simulink model "vdp_1_mode"  (R2020a)
settings: Solver=VariableStepAuto  StartTime=0.0  StopTime=60  RelTol=1e-3
libraries: dspsnks4 x1
settings Model: EnablePacing=on  Creator=Dinh-Viet-Toan  LastModifiedBy=Dinh-Viet-Toan

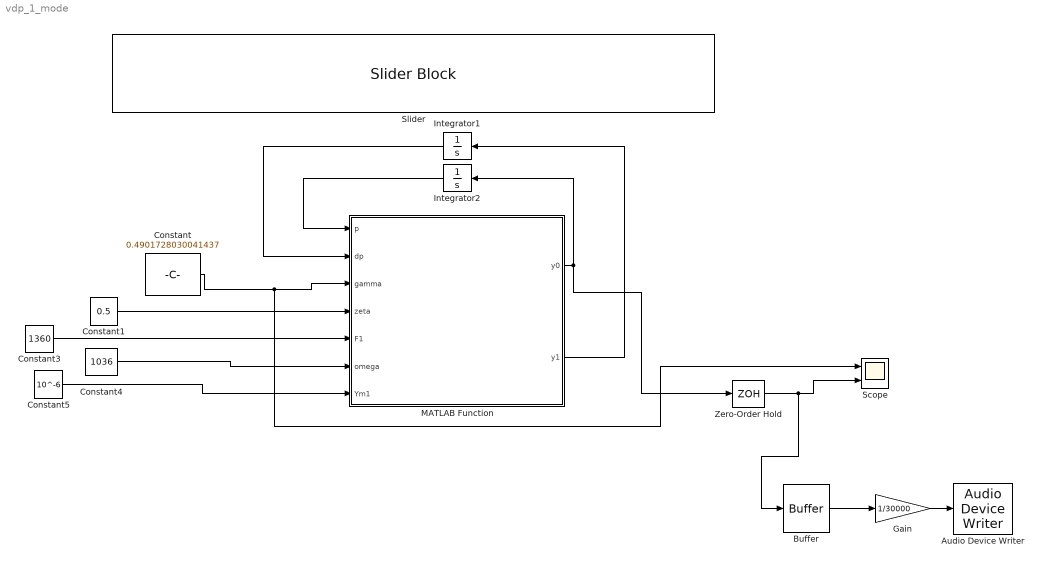
== system vdp_1_mode ==
  Audio Device Writer : dspsnks4/Audio Device Writer  Driver=DirectSound  Device=Default  InheritSampleRate=on  SampleRate=44100  BitDepth=16-bit integer  BufferSize=4096  NumBuffers=10  DefaultOutputChannelMapping=on  OutputChannelMapping=1:2  OutputNumUnderrunSamples=off  DriverIdx=1  DeviceWarnFlag=''
  Buffer : Buffer  N=10000  V=1024  OutputFrames=off
  Constant : Constant  Value=0.4901728030041437
  Constant1 : Constant  Value=0.5
  Constant3 : Constant  Value=1360
  Constant4 : Constant  Value=1036
  Constant5 : Constant  Value=10^-6
  Gain : Gain  Gain=1/30000
  Integrator1 : Integrator
  Integrator2 : Integrator  InitialCondition=0.01
  MATLAB Function : MATLAB Function  TreatAsAtomicUnit=on
  Scope : Scope  NumInputPorts=2
  Slider : SliderBlock  ScaleMin=0.001  ScaleMax=1
  Zero-Order Hold : ZeroOrderHold  SampleTime=1/22050
  wires:
  Constant/1 -> Scope/1, MATLAB Function/3(gamma)
  Constant3/1 -> MATLAB Function/5(F1)
  Constant4/1 -> MATLAB Function/6(omega)
  Constant5/1 -> MATLAB Function/7(Ym1)
  Integrator1/1 -> MATLAB Function/2(dp)
  MATLAB Function/2(y1) -> Integrator1/1
  Integrator2/1 -> MATLAB Function/1(p)
  Constant1/1 -> MATLAB Function/4(zeta)
  MATLAB Function/1(y0) -> Zero-Order Hold/1, Integrator2/1
  Zero-Order Hold/1 -> Buffer/1, Scope/2
  Buffer/1 -> Gain/1
  Gain/1 -> Audio Device Writer/1

== matlab function vdp_1_mode/MATLAB Function ==
  data: p input; y0 output; dp input; gamma input; zeta input; F1 input; omega input; Ym1 input; y1 output
function [y0, y1] = fcn(p, dp, gamma, zeta,F1, omega, Ym1)

A = zeta * (3*gamma-1)/(2*sqrt(gamma));
B = -zeta*(3*gamma+1) / (8*gamma^(3/2));
C = -zeta*(gamma+1)/(16*gamma^(5/2));

y0 = dp;
y1 = -F1*((Ym1-A) - 2*B*p - 3*C*p^2)*dp - p*omega^2;
